simulink model "Signal2"  (Simulink 9.1)
settings: Solver=ode45  StartTime=0.0  StopTime=10.0  RelTol=1e-3  EnableMultiTasking=on
settings Model: Creator=Admin  LastModifiedBy=Asus
settings DataIOCC: LimitDataPoints=on  SignalLoggingSaveFormat=ModelDataLogs
settings OptimizationCC: ExpressionDepthLimit=2147483647
settings DebuggingCC: SolverPrmCheckMsg=warning  FcnCallInpInsideContextMsg=warning  StateNameClashWarn=warning
settings GRTTargetCC: GeneratePreprocessorConditionals=Disable all  CombineOutputUpdateFcns=on  GRTInterface=off

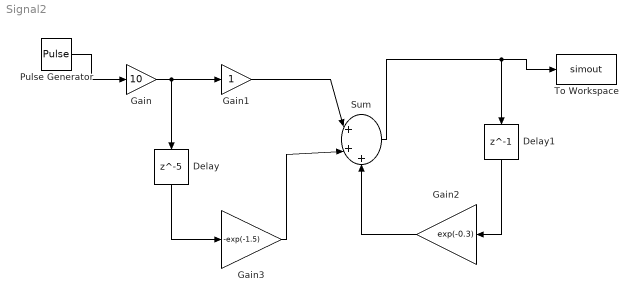
== system Signal2 ==
  Delay : Delay  DelayLength=5
  Delay1 : Delay  DelayLength=1
  Gain : Gain  Gain=10
  Gain1 : Gain
  Gain2 : Gain  Gain=exp(-0.3)
  Gain3 : Gain  Gain=-exp(-1.5)
  Pulse Generator : DiscretePulseGenerator  Period=100
  Sum : Sum  Inputs=|+++
  To Workspace : ToWorkspace  VariableName=simout  SampleTime=-1
  wires:
  Gain3/1 -> Sum/2
  Delay/1 -> Gain3/1
  Gain/1 -> Gain1/1, Delay/1
  Gain1/1 -> Sum/1
  Delay1/1 -> Gain2/1
  Gain2/1 -> Sum/3
  Sum/1 -> Delay1/1, To Workspace/1
  Pulse Generator/1 -> Gain/1
